simulink library "library_mpc"  (R2016b)
settings: Solver=VariableStepAuto  StartTime=0.0  StopTime=10.0  RelTol=1e-3
settings Model: Creator=jgillis  LastModifiedBy=jgillis

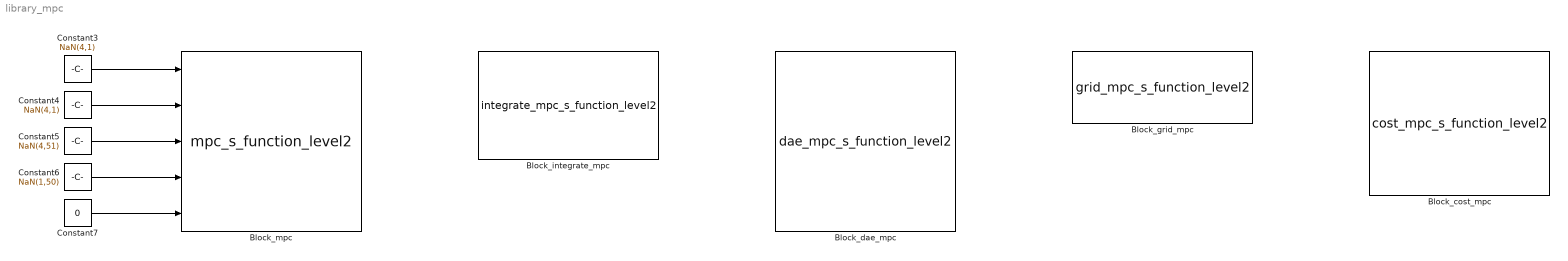
== system library_mpc ==
  Block_mpc : S-Function  FunctionName=mpc_s_function_level2  SFunctionDeploymentMode=off  EnableBusSupport=off  InitFcn=|  SFunctionModules='mpc_codegen mpc'
      | solver_stats_bus = Simulink.Bus;
      | elements = {};
      | e = Simulink.BusElement;
      | e.Name = 'sqp_stop_crit';
      | e.DataType = 'int32';
      | elements{end+1} = e;
      | e = Simulink.BusElement;
      | e.Name = 'n_sqp_iter';
      | e.DataType = 'int32';
      | elements{end+1} = e;
      | e = Simulink.BusElement;
      | e.Name = 'n_ls';
      | e.DataType = 'int32';
      | elements{end+1} = e;
      | e = Simulink.BusElement;
      | e.Name = 'n_max_ls';
      | e.DataType = 'int32';
      | elements{end+1} = e;
      | e = Simulink.BusElement;
      | e.Name = 'n_qp_iter';
      | e.DataType = 'int32';
      | elements{end+1} = e;
      | e = Simulink.BusElement;
      | e.Name = 'n_max_qp_iter';
      | e.DataType = 'int32';
      | elements{end+1} = e;
      | e = Simulink.BusElement;
      | e.Name = 'runtime';
      | e.DataType = 'double';
      | elements{end+1} = e;
      | solver_stats_bus.Elements = [elements{:}];
      mask Display:
      | port_label('input',1,'x_current');
      | port_label('input',2,'x_final');
      | port_label('input',3,'x_initial_guess');
      | port_label('input',4,'u_initial_guess');
      | port_label('input',5,'hotstart');
      | disp('IMPACT MPC\nmpc');
      | port_label('output',1,'x_opt @ k=1');
      | port_label('output',2,'u_opt @ k=0');
      | port_label('output',3,'solver stats');
  Constant3 : Constant  Value=NaN(4,1)  VectorParams1D=off
  Constant4 : Constant  Value=NaN(4,1)  VectorParams1D=off
  Constant5 : Constant  Value=NaN(4,51)  VectorParams1D=off
  Constant6 : Constant  Value=NaN(1,50)  VectorParams1D=off
  Constant7 : Constant  Value=0  VectorParams1D=off
  Block_integrate_mpc : S-Function  FunctionName=integrate_mpc_s_function_level2  SFunctionDeploymentMode=off  EnableBusSupport=off
      mask Display:
      | port_label('input',1,'x');
      | port_label('input',2,'u');
      | port_label('input',3,'dt');
      | disp('integrate_mpc');
      | port_label('output',1,'xf');
  Block_dae_mpc : S-Function  FunctionName=dae_mpc_s_function_level2  SFunctionDeploymentMode=off  EnableBusSupport=off
      mask Display:
      | port_label('input',1,'x');
      | port_label('input',2,'u');
      | port_label('input',3,'z');
      | port_label('input',4,'p');
      | port_label('input',5,'t');
      | disp('dae_mpc');
      | port_label('output',1,'ode');
      | port_label('output',2,'alg');
  Block_grid_mpc : S-Function  FunctionName=grid_mpc_s_function_level2  SFunctionDeploymentMode=off  EnableBusSupport=off
      mask Display:
      | port_label('input',1,'x_current');
      | port_label('input',2,'x_final');
      | disp('grid_mpc');
      | port_label('output',1,'grid');
  Block_cost_mpc : S-Function  FunctionName=cost_mpc_s_function_level2  SFunctionDeploymentMode=off  EnableBusSupport=off
      mask Display:
      | port_label('input',1,'x');
      | port_label('input',2,'u');
      | port_label('input',3,'x_current');
      | port_label('input',4,'x_final');
      | disp('cost_mpc');
      | port_label('output',1,'f');
  wires:
  Constant3/1 -> Block_mpc/1
  Constant4/1 -> Block_mpc/2
  Constant5/1 -> Block_mpc/3
  Constant6/1 -> Block_mpc/4
  Constant7/1 -> Block_mpc/5
